simulink model "inverter_switching_GridFollowing_StudentVersion"  (R2025a)
settings: Solver=ode1be  StartTime=0.0  StopTime=0.2  FixedStep=1e-6  MaxStep=1e-7  RelTol=1e-3
values from neighbouring files (symbols this model uses):
  C_Filter = 300e-6    (= 0.0003)    [parameters_StudentVersion.m]
  kFilterIdq = wnFiltreIdq/WnIdq    (= 1)    [parameters_StudentVersion.m]
  kFilterVdq = wnFiltreVdq/WnVdq    (= 1)    [parameters_StudentVersion.m]
  Kpll2 = 1    [parameters_StudentVersion.m]
  L_Filter = 1e-3    (= 0.001)    [parameters_StudentVersion.m]
  rL_filter = 0.1    [parameters_StudentVersion.m]
  T1 = 10/wcpll    (= 10)    [parameters_StudentVersion.m]
  T2 = 1/(10*wcpll)    (= 0.1)    [parameters_StudentVersion.m]
  T32 = sqrt(2/3)*[1 0; -1/2 sqrt(3)/2; -1/2 -sqrt(3)/2]    [parameters_StudentVersion.m]
  Ts = 1/Fs    (= 5e-05)    [parameters_StudentVersion.m]
  Vdc = 800    [parameters_StudentVersion.m]
  Vrms_Grid = 110    [parameters_StudentVersion.m]
  WnIdq = 12000    [parameters_StudentVersion.m]
  WnVdq = 1200    [parameters_StudentVersion.m]
  wrated = 2*pi*60    (= 376.991118431)    [parameters_StudentVersion.m]
  zeta = 1/sqrt(2)    [parameters_StudentVersion.m]
undefined symbols (not defined in the file or in its folder): DiscIntNeverNeededParam
libraries: nesl_utility x22, ee_lib x16, fl_lib x15, simulink x3
(part 1 of 2)
settings Model: Creator=bahrami1  LastModifiedBy=bahrami1

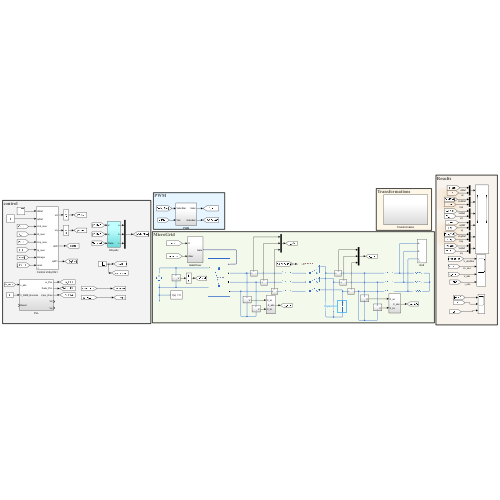
[thumbnail: Simulink's stored preview of the top-level diagram]
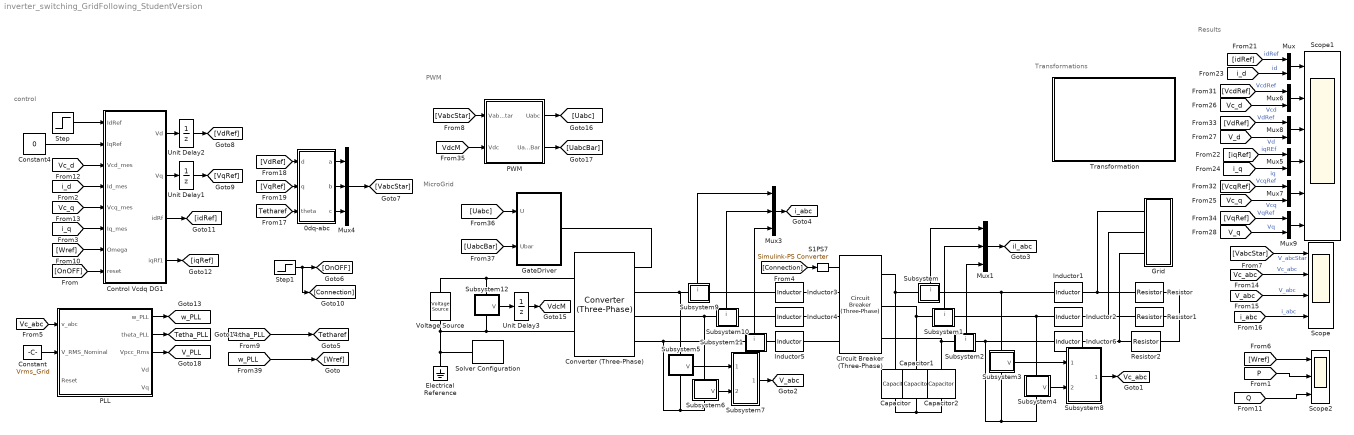
== system inverter_switching_GridFollowing_StudentVersion ==
  note: Transformations
  note: control
  note: MicroGrid
  note: Results
  note: PWM
  0dq-abc : Subsystem
  Capacitor : ee_lib/Passive/Capacitor  cap_option=ee.enum.passive.capacitor.capOption.const  c=10e-6 F  Cvec=[1e-05, 1e-06] F  Vvec=[0, 10] V  CV_table_symmetry=ee.enum.passive.capacitor.tableSymmetry.yes  f_vec=[1, 10] kHz  DFext_vec=[.8, 1.2]  enable_C_tol=ee.enum.toleranceApplication.none  averaging_period=0 s  C_tol=5  tol_distribution=ee.enum.toleranceDistribution.uniform  nSigma=4  r=0 Ohm  g=0 1/Ohm  enable_operating_limits=ee.enum.enable.no  operating_limit_action=ee.enum.passive.reportOpLim.warn  max_working_voltage_range=[-25, 25] V  power_rating=1 W  maxTemperature=85 degC  thermalEnable=false  thermalMass=1 J/K  i_specify=off  i_priority=None  i=0 A  i_nominal_specify=off  i_nominal_value=1  i_nominal_unit=A  v_specify=on  v_priority=None  v=Vrms_Grid*cos(0) V  v_nominal_specify=off  v_nominal_value=1  v_nominal_unit=V  vc_specify=on  vc_priority=High  vc=Vrms_Grid*cos(0) V  vc_nominal_specify=off  vc_nominal_value=1  vc_nominal_unit=V  T_specify=off  T_priority=None  T=298.15 K  T_nominal_specify=off  T_nominal_value=1  T_nominal_unit=K
  Capacitor1 : ee_lib/Passive/Capacitor  cap_option=ee.enum.passive.capacitor.capOption.const  c=10e-6 F  Cvec=[1e-05, 1e-06] F  Vvec=[0, 10] V  CV_table_symmetry=ee.enum.passive.capacitor.tableSymmetry.yes  f_vec=[1, 10] kHz  DFext_vec=[.8, 1.2]  enable_C_tol=ee.enum.toleranceApplication.none  averaging_period=0 s  C_tol=5  tol_distribution=ee.enum.toleranceDistribution.uniform  nSigma=4  r=0 Ohm  g=0 1/Ohm  enable_operating_limits=ee.enum.enable.no  operating_limit_action=ee.enum.passive.reportOpLim.warn  max_working_voltage_range=[-25, 25] V  power_rating=1 W  maxTemperature=85 degC  thermalEnable=false  thermalMass=1 J/K  i_specify=off  i_priority=None  i=0 A  i_nominal_specify=off  i_nominal_value=1  i_nominal_unit=A  v_specify=on  v_priority=None  v=Vrms_Grid*cos(-2*pi/3) V  v_nominal_specify=off  v_nominal_value=1  v_nominal_unit=V  vc_specify=on  vc_priority=High  vc=Vrms_Grid*cos(-2*pi/3) V  vc_nominal_specify=off  vc_nominal_value=1  vc_nominal_unit=V  T_specify=off  T_priority=None  T=298.15 K  T_nominal_specify=off  T_nominal_value=1  T_nominal_unit=K
  Capacitor2 : ee_lib/Passive/Capacitor  cap_option=ee.enum.passive.capacitor.capOption.const  c=10e-6 F  Cvec=[1e-05, 1e-06] F  Vvec=[0, 10] V  CV_table_symmetry=ee.enum.passive.capacitor.tableSymmetry.yes  f_vec=[1, 10] kHz  DFext_vec=[.8, 1.2]  enable_C_tol=ee.enum.toleranceApplication.none  averaging_period=0 s  C_tol=5  tol_distribution=ee.enum.toleranceDistribution.uniform  nSigma=4  r=0 Ohm  g=0 1/Ohm  enable_operating_limits=ee.enum.enable.no  operating_limit_action=ee.enum.passive.reportOpLim.warn  max_working_voltage_range=[-25, 25] V  power_rating=1 W  maxTemperature=85 degC  thermalEnable=false  thermalMass=1 J/K  i_specify=off  i_priority=None  i=0 A  i_nominal_specify=off  i_nominal_value=1  i_nominal_unit=A  v_specify=on  v_priority=None  v=Vrms_Grid*cos(+2*pi/3) V  v_nominal_specify=off  v_nominal_value=1  v_nominal_unit=V  vc_specify=on  vc_priority=High  vc=Vrms_Grid*cos(+2*pi/3) V  vc_nominal_specify=off  vc_nominal_value=1  vc_nominal_unit=V  T_specify=off  T_priority=None  T=298.15 K  T_nominal_specify=off  T_nominal_value=1  T_nominal_unit=K
  Circuit Breaker (Three-Phase) : ee_lib/Switches & Breakers/Circuit Breaker (Three-Phase)  R_closed=1e-9 Ohm  G_open=1e-12 1/Ohm  threshold=0.5 V  breaker_behavior=ee.enum.switches.breakerBehavior.zeroCrossingDisable
      settings: InternalSimscapePortConfiguration="{\"Bottom\":[],\"Left\":[{\"id\":\"vT\",\"label\":\"vT\",\"type\":\"input\"},{\"id\":\"a1\",\"label\":\"a1\",\"type\":\"foundation.electrical.electrical\"},{\"id\":\"b1\",\"label\":\"b1\",\"type\":\"foundation.electrical.electrical\"},{\"id\":\"c1\",\"label\":\"c1\",\"type\":\"foundation.electrical.electrical\"}],\"Right\":[{\"id\":\"a2\",\"label\":\"a2\",\"type\":\"foundation.electrical.electrical\"},{\"id\":\"b2\",\"label\":\"b2\",\"type\":\"foundation.electrical.electrical\"},{\"id\":\"c2\",\"label\":\"c2\",\"type\":\"foundation.electrical.electrical\"}],\"Top\":[]}"
  Constant : Constant  Value=Vrms_Grid
  Constant4 : Constant  Value=0
  Control Vcdq DG1 : Subsystem  mask{rL_DG=rL_filter, L_DG=L_Filter, C_DG=C_Filter, Wn_Idq=WnIdq, kFilter_Idq=kFilterIdq, IntegIdLimitNeg=-30000/L_Filter, IntegIdLimitPos=30000/L_Filter, IntegIqLimitNeg=-30000/L_Filter, IntegIqLimitPos=30000/L_Filter, Wn_Vdq=WnVdq, kFilter_Vdq=kFilterVdq, idRef_Min=-500, idRef_Max=500, iqRef_Min=-500, iqRef_Max=500}
      mask prompts: rL_DG "rl_DG :"; L_DG "L_DG :"; C_DG "C_DG :"; Wn_Idq "Wn_Idq :"; kFilter_Idq "kFilter_Idq :"; Wn_Vdq "Wn_Vdq :"; kFilter_Vdq "kFilter Vdq :"; idRef_Min "idRef_Min :"; idRef_Max "idRef_Max :"; iqRef_Min "iqRef_Min :"; iqRef_Max "iqRef_Max :"
      mask DialogControl ControlGroupParameters Prompt: Control
      mask DialogControl SaturationGroup Prompt: Saturation
  Converter (Three-Phase) : ee_lib/Semiconductors & Converters/Converters/Converter (Three-Phase)  port_option=ee.enum.threePhasePort.expanded  fidelity_option=ee.enum.converters.fidelity.detailed  device_type=ee.enum.converters.switchingdevice.averaged  showThermalPort=false  K=0  Vth=6 V  Vgt=1 V  Vgt_off=-1 V  Ih=1 A  Vf=0.8 V  Ron=0.001 Ohm  Rds=0.001 Ohm  Goff=1e-6 1/Ohm  Eon_scalar=22.86e-3 J  Eoff_scalar=17.14e-3 J  Eoff_natural_commutation=10e-3 J  Voff=300 V  Iout_scalar=600 A  onCurrentMeasDelay=0 s  useCurrentFromPreviousCycle=false  useVoltageFromPreviousCycle=false  diode_param=ee.enum.converters.protectiondiode.chargedynamics  diode_Vf=0.8 V  diode_Ron=0.001 Ohm  diode_Goff=1e-5 1/Ohm  diode_C=50 nF  diode_iRM=-235 A  diode_iF=300 A  diode_idot=-50 A/us  diode_trr_param=ee.enum.converters.diodetrr.trr_factor  diode_trr_factor=3  diode_trr=15 us  diode_Qrr=1500 s*uA  diode_rec_loss_model=ee.enum.diode.reverseRecoveryModel.fixed  diode_ErecVal=0 J  diode_scaleWithIandV=false  diode_ErecMat=zeros(2, 3) J  diode_TjrecVec=[298.15, 398.15] K  diode_IfrecVec=[.1, 1, 10] A  diode_IrecVal=10 A  diode_VrecVal=10 V  diode_tFilter=1 / 1000 / 100 s  thermal_network_parameterization=ee.enum.thermalNetworkTopology.external  Rth=[.08, .5] K/W  Rth_Cauer=[.08, .1, .5] K/W  Rth_Foster=[.08, .14, .22, .16] K/W  thermal_mass_parameterization=ee.enum.thermalNetwork.timeconstant  thermal_mass=[.01, .5] J/K  thermal_mass_Cauer=[.01, .1, .5] J/K  thermal_mass_Foster=[.001, .005, .05, .5] J/K  thermal_time_constant=[.001, .2] s  thermal_time_constant_Cauer=[.001, .1, .2] s  thermal_time_constant_Foster=[7e-05, .0007, .01, .08] s  thermal_mass_initial_temperatures=[25, 25] degC  thermal_mass_initial_temperatures_Cauer=[25, 25, 25] degC  junction_thermal_mass=0.01 J/K  Tvec_initial_Foster=[25, 25, 25, 25] degC  snubber_type=ee.enum.converters.snubber.exclude  Cs=1e-7 F  Rs=0.1 Ohm  Vce_loss=[0, 150, 300] V
      settings: InternalSimscapePortConfiguration="{\"Bottom\":[],\"Left\":[{\"id\":\"G\",\"label\":\"G\",\"type\":\"foundation.electrical.twelve_phase\"},{\"id\":\"a\",\"label\":\"a\",\"type\":\"foundation.electrical.electrical\"},{\"id\":\"b\",\"label\":\"b\",\"type\":\"foundation.electrical.electrical\"},{\"id\":\"c\",\"label\":\"c\",\"type\":\"foundation.electrical.electrical\"}],\"Right\":[{\"id\":\"p\",\"label\":\"+\",\"type\":\"foundation.electrical.electrical\"},{\"id\":\"n\",\"label\":\"-\",\"type\":\"foundation.electrical.electrical\"}],\"Top\":[]}"
  Electrical Reference : fl_lib/Electrical/Electrical Elements/Electrical Reference
  GateDriver : Subsystem
  Grid : Subsystem  mask{Vrms_Grid=Vrms_Grid, F_Grid=60, Phase_Grid=0}
      mask prompts: Vrms_Grid "Grid Voltage (RMS):"; F_Grid "Grid Frequency:"; Phase_Grid "Grid phase angle:"
  Inductor1 : ee_lib/Passive/Inductor  l=1e-3 H  enable_L_tol=ee.enum.toleranceApplication.none  L_tol=20  tol_distribution=ee.enum.toleranceDistribution.uniform  nSigma=4  r=0.5 Ohm  g=1e-9 1/Ohm  enable_operating_limits=ee.enum.enable.no  operating_limit_action=ee.enum.passive.reportOpLim.warn  max_working_current=1 A  power_rating=1 W  i_L_specify=off  i_L_priority=High  i_L=0 A  i_L_nominal_specify=off  i_L_nominal_value=1  i_L_nominal_unit=A
  Inductor2 : ee_lib/Passive/Inductor  l=1e-3 H  enable_L_tol=ee.enum.toleranceApplication.none  L_tol=20  tol_distribution=ee.enum.toleranceDistribution.uniform  nSigma=4  r=0.5 Ohm  g=1e-9 1/Ohm  enable_operating_limits=ee.enum.enable.no  operating_limit_action=ee.enum.passive.reportOpLim.warn  max_working_current=1 A  power_rating=1 W  i_L_specify=off  i_L_priority=High  i_L=0 A  i_L_nominal_specify=off  i_L_nominal_value=1  i_L_nominal_unit=A
  Inductor3 : ee_lib/Passive/Inductor  l=10e-3 H  enable_L_tol=ee.enum.toleranceApplication.none  L_tol=20  tol_distribution=ee.enum.toleranceDistribution.uniform  nSigma=4  r=0 Ohm  g=1e-9 1/Ohm  enable_operating_limits=ee.enum.enable.no  operating_limit_action=ee.enum.passive.reportOpLim.warn  max_working_current=1 A  power_rating=1 W  i_L_specify=off  i_L_priority=High  i_L=0 A  i_L_nominal_specify=off  i_L_nominal_value=1  i_L_nominal_unit=A
  Inductor4 : ee_lib/Passive/Inductor  l=10e-3 H  enable_L_tol=ee.enum.toleranceApplication.none  L_tol=20  tol_distribution=ee.enum.toleranceDistribution.uniform  nSigma=4  r=0 Ohm  g=1e-9 1/Ohm  enable_operating_limits=ee.enum.enable.no  operating_limit_action=ee.enum.passive.reportOpLim.warn  max_working_current=1 A  power_rating=1 W  i_L_specify=off  i_L_priority=High  i_L=0 A  i_L_nominal_specify=off  i_L_nominal_value=1  i_L_nominal_unit=A
  Inductor5 : ee_lib/Passive/Inductor  l=10e-3 H  enable_L_tol=ee.enum.toleranceApplication.none  L_tol=20  tol_distribution=ee.enum.toleranceDistribution.uniform  nSigma=4  r=0 Ohm  g=1e-9 1/Ohm  enable_operating_limits=ee.enum.enable.no  operating_limit_action=ee.enum.passive.reportOpLim.warn  max_working_current=1 A  power_rating=1 W  i_L_specify=off  i_L_priority=High  i_L=0 A  i_L_nominal_specify=off  i_L_nominal_value=1  i_L_nominal_unit=A
  Inductor6 : ee_lib/Passive/Inductor  l=1e-3 H  enable_L_tol=ee.enum.toleranceApplication.none  L_tol=20  tol_distribution=ee.enum.toleranceDistribution.uniform  nSigma=4  r=0.5 Ohm  g=1e-9 1/Ohm  enable_operating_limits=ee.enum.enable.no  operating_limit_action=ee.enum.passive.reportOpLim.warn  max_working_current=1 A  power_rating=1 W  i_L_specify=off  i_L_priority=High  i_L=0 A  i_L_nominal_specify=off  i_L_nominal_value=1  i_L_nominal_unit=A
  Mux{,5..9} (6 alike) : Mux  Inputs=2
  Mux1 : Mux  Inputs=3
  Mux3 : Mux  Inputs=3
  Mux4 : Mux  Inputs=3
  PLL : Subsystem
  PWM : Subsystem
  Resistor : ee_lib/Passive/Resistor  R=5 Ohm  enable_R_tol=ee.enum.toleranceApplication.none  R_tol=5  tol_distribution=ee.enum.toleranceDistribution.uniform  nSigma=4  enable_operating_limits=ee.enum.enable.no  operating_limit_action=ee.enum.passive.reportOpLim.warn  power_rating=1 W  max_working_voltage=100 V  noise_mode=ee.enum.sources.noise.Disabled  Tdevice=25 degC  sample_time=1e-3 s  repeatability=ee.enum.ic.repeatability.notRepeatable  user_seed=0  auto_seed=3890346746  power_derating_T1=70 degC  power_derating_T2=155 degC  operating_temperature_range_vec=[-50, 150] degC  alpha=3.93e-3 1/K  Tmeas=25 degC  thermal_mass=100 J/K  temperature_specify=off  temperature_priority=High  temperature=298.15 K  temperature_nominal_specify=off  temperature_nominal_value=1  temperature_nominal_unit=K
  Resistor1 : ee_lib/Passive/Resistor  R=5 Ohm  enable_R_tol=ee.enum.toleranceApplication.none  R_tol=5  tol_distribution=ee.enum.toleranceDistribution.uniform  nSigma=4  enable_operating_limits=ee.enum.enable.no  operating_limit_action=ee.enum.passive.reportOpLim.warn  power_rating=1 W  max_working_voltage=100 V  noise_mode=ee.enum.sources.noise.Disabled  Tdevice=25 degC  sample_time=1e-3 s  repeatability=ee.enum.ic.repeatability.notRepeatable  user_seed=0  auto_seed=545404223  power_derating_T1=70 degC  power_derating_T2=155 degC  operating_temperature_range_vec=[-50, 150] degC  alpha=3.93e-3 1/K  Tmeas=25 degC  thermal_mass=100 J/K  temperature_specify=off  temperature_priority=High  temperature=298.15 K  temperature_nominal_specify=off  temperature_nominal_value=1  temperature_nominal_unit=K
  Resistor2 : ee_lib/Passive/Resistor  R=5 Ohm  enable_R_tol=ee.enum.toleranceApplication.none  R_tol=5  tol_distribution=ee.enum.toleranceDistribution.uniform  nSigma=4  enable_operating_limits=ee.enum.enable.no  operating_limit_action=ee.enum.passive.reportOpLim.warn  power_rating=1 W  max_working_voltage=100 V  noise_mode=ee.enum.sources.noise.Disabled  Tdevice=25 degC  sample_time=1e-3 s  repeatability=ee.enum.ic.repeatability.notRepeatable  user_seed=0  auto_seed=3922919431  power_derating_T1=70 degC  power_derating_T2=155 degC  operating_temperature_range_vec=[-50, 150] degC  alpha=3.93e-3 1/K  Tmeas=25 degC  thermal_mass=100 J/K  temperature_specify=off  temperature_priority=High  temperature=298.15 K  temperature_nominal_specify=off  temperature_nominal_value=1  temperature_nominal_unit=K
  S1PS7 : nesl_utility/Simulink-PS Converter  PhysicalDomain=network_engine_domain  SubClassName=ps_input  LeftPortType=input  RightPortType=output  PseudoPeriodic=off  Frequencies=[]  NoiseDistribution=none  NoiseParameters=[]  Unit=1  AffineConversion=off  FilteringAndDerivatives=zero  SimscapeFilterOrder=1  InputFilterTimeConstant=.001  UdotUserProvided=1
  Scope : Scope  NumInputPorts=4
      settings: ActiveDisplayString=4  ActiveDisplayYMinimum=-4.8438387041910405  ActiveDisplayYMaximum=5.5775843218677732
  Scope1 : Scope  NumInputPorts=6
      settings: ActiveDisplayString=6  ActiveDisplayYMinimum=-764.96979422436971  ActiveDisplayYMaximum=755.2359372195092
  Scope2 : Scope  NumInputPorts=3
      settings: ActiveDisplayYMinimum=-44.93774115699739  ActiveDisplayYMaximum=222.58045892307609  DataLoggingVariableName=ScopeData2
  Solver Configuration : nesl_utility/Solver Configuration  PhysicalDomain=network_engine_domain  SubClassName=solver  LeftPortType=input  RightPortType=generic  Tones=[]  Harmonics=[]  SimulateNoise=off  Profile=off  UseLocalSampling=off  EnableSwitchedLinearOptims=on  FrequencyDomain=off  UseCCode=off  RelTol=0.001  AbsTol=0.001  MinStep=1e-09  ToWorkspace=off  RevertToSquareIcSolve=off  NumHomotopyIterations=100  PhasorMode=off  PhasorModeNumHarmonics=1  ConsistencySolver=NEWTON_XTOL_AFTER_FTOL  IndexReductionMethod=DerivativeReplacement  DoDC=off  ResidualTolerance=1e-09  ConsistencyTolSource=GLOBAL  ConsistencyAbsTol=0.001  ConsistencyRelTol=0.001  ConsistencyTolFactor=1e-9  UseLocalSolver=off  LocalSolverChoice=NE_PARTITIONING_ADVANCER  ResolveIndetEquations=on  FunctionEvalNumThread=1  LocalSolverSampleTime=50e-6  DoFixedCost=on  MaxNonlinIter=3  MaxModeIter=2  ComputeImpulses=off  ImpulseIterations=2  LinearAlgebra=auto  LinearAlgebraNumThread=0  EquationFormulation=NE_TIME_EF  DelaysMemoryBudget=1024  AutomaticFiltering=on  FilteringTimeConstant=0.001  PartitionStorageMethod=AS_NEEDED  PartitionMemoryBudget=1024  PartitionMethod=ROBUST  MultibodyUseLocalSolver=off  MultibodyLocalSolverChoice=ODE1  MultibodyLocalSolverSampleTime=0.001
  Step : Step  Time=0.04  After=4  SampleTime=0
  Step1 : Step  Time=0.02  Before=1  After=0  SampleTime=0
  Subsystem : Subsystem
      settings: PortSchema="{\"entries\":[{\"content\":{\"sides\":[{\"content\":{\"connectorIds\":[\"LConn1\"]},\"type\":\"ConnectorPlacement.EquallySpacedRectSide\",\"uuid\":\"f9dae77b-82ec-46c0-8ec7-07c4c343cd61\"},{\"content\":{\"connectorIds\":[\"RConn1\"],\"side\":\"RIGHT\"},\"type\":\"ConnectorPlacement.EquallySpacedRectSide\",\"uuid\":\"c868f1e8-59aa-45a3-abdf-5b79dca1cbd6\"},{\"content\":{\"connectorIds\":[\"Out1\"],\"side\":\"TOP\"},\"type\":\"ConnectorPlacement.EquallySpacedRectSide\",\"uuid\":\"1fe3fd4f-ec18-4909-aef2-795910f5eee8\"}]},\"type\":\"ConnectorPlacement.EquallySpacedConnector\",\"uuid\":\"b65f0ac3-40cf-4bf8-a5c1-5ed6a13721a4\"}],\"packageUris\":[\"http://schema.mathworks.com/mf0/Connector/R2020b\"],\"version\":\"1.0\"}"
  Subsystem1 : Subsystem
      settings: PortSchema="{\"entries\":[{\"content\":{\"sides\":[{\"content\":{\"connectorIds\":[\"LConn1\"]},\"type\":\"ConnectorPlacement.EquallySpacedRectSide\",\"uuid\":\"f9dae77b-82ec-46c0-8ec7-07c4c343cd61\"},{\"content\":{\"connectorIds\":[\"RConn1\"],\"side\":\"RIGHT\"},\"type\":\"ConnectorPlacement.EquallySpacedRectSide\",\"uuid\":\"c868f1e8-59aa-45a3-abdf-5b79dca1cbd6\"},{\"content\":{\"connectorIds\":[\"Out1\"],\"side\":\"TOP\"},\"type\":\"ConnectorPlacement.EquallySpacedRectSide\",\"uuid\":\"1fe3fd4f-ec18-4909-aef2-795910f5eee8\"}]},\"type\":\"ConnectorPlacement.EquallySpacedConnector\",\"uuid\":\"b65f0ac3-40cf-4bf8-a5c1-5ed6a13721a4\"}],\"packageUris\":[\"http://schema.mathworks.com/mf0/Connector/R2020b\"],\"version\":\"1.0\"}"
  Subsystem10 : Subsystem
      settings: PortSchema="{\"entries\":[{\"content\":{\"sides\":[{\"content\":{\"connectorIds\":[\"LConn1\"]},\"type\":\"ConnectorPlacement.EquallySpacedRectSide\",\"uuid\":\"f9dae77b-82ec-46c0-8ec7-07c4c343cd61\"},{\"content\":{\"connectorIds\":[\"RConn1\"],\"side\":\"RIGHT\"},\"type\":\"ConnectorPlacement.EquallySpacedRectSide\",\"uuid\":\"c868f1e8-59aa-45a3-abdf-5b79dca1cbd6\"},{\"content\":{\"connectorIds\":[\"Out1\"],\"side\":\"TOP\"},\"type\":\"ConnectorPlacement.EquallySpacedRectSide\",\"uuid\":\"1fe3fd4f-ec18-4909-aef2-795910f5eee8\"}]},\"type\":\"ConnectorPlacement.EquallySpacedConnector\",\"uuid\":\"b65f0ac3-40cf-4bf8-a5c1-5ed6a13721a4\"}],\"packageUris\":[\"http://schema.mathworks.com/mf0/Connector/R2020b\"],\"version\":\"1.0\"}"
  Subsystem11 : Subsystem
      settings: PortSchema="{\"entries\":[{\"content\":{\"sides\":[{\"content\":{\"connectorIds\":[\"LConn1\"]},\"type\":\"ConnectorPlacement.EquallySpacedRectSide\",\"uuid\":\"f9dae77b-82ec-46c0-8ec7-07c4c343cd61\"},{\"content\":{\"connectorIds\":[\"RConn1\"],\"side\":\"RIGHT\"},\"type\":\"ConnectorPlacement.EquallySpacedRectSide\",\"uuid\":\"c868f1e8-59aa-45a3-abdf-5b79dca1cbd6\"},{\"content\":{\"connectorIds\":[\"Out1\"],\"side\":\"TOP\"},\"type\":\"ConnectorPlacement.EquallySpacedRectSide\",\"uuid\":\"1fe3fd4f-ec18-4909-aef2-795910f5eee8\"}]},\"type\":\"ConnectorPlacement.EquallySpacedConnector\",\"uuid\":\"b65f0ac3-40cf-4bf8-a5c1-5ed6a13721a4\"}],\"packageUris\":[\"http://schema.mathworks.com/mf0/Connector/R2020b\"],\"version\":\"1.0\"}"
  Subsystem12 : Subsystem
      settings: PortSchema="{\"entries\":[{\"content\":{\"sides\":[{\"content\":{},\"type\":\"ConnectorPlacement.EquallySpacedRectSide\",\"uuid\":\"f9dae77b-82ec-46c0-8ec7-07c4c343cd61\"},{\"content\":{\"connectorIds\":[\"Out1\"],\"side\":\"RIGHT\"},\"type\":\"ConnectorPlacement.EquallySpacedRectSide\",\"uuid\":\"c868f1e8-59aa-45a3-abdf-5b79dca1cbd6\"},{\"content\":{\"connectorIds\":[\"LConn1\"],\"side\":\"TOP\"},\"type\":\"ConnectorPlacement.EquallySpacedRectSide\",\"uuid\":\"1fe3fd4f-ec18-4909-aef2-795910f5eee8\"},{\"content\":{\"connectorIds\":[\"RConn1\"],\"side\":\"BOTTOM\"},\"type\":\"ConnectorPlacement.EquallySpacedRectSide\",\"uuid\":\"67a88f15-4497-4048-9449-885deab38afe\"}]},\"type\":\"ConnectorPlacement.EquallySpacedConnector\",\"uuid\":\"b65f0ac3-40cf-4bf8-a5c1-5ed6a13721a4\"}],\"packageUris\":[\"http://schema.mathworks.com/mf0/Connector/R2020b\"],\"version\":\"1.0\"}"
  Subsystem2 : Subsystem
      settings: PortSchema="{\"entries\":[{\"content\":{\"sides\":[{\"content\":{\"connectorIds\":[\"LConn1\"]},\"type\":\"ConnectorPlacement.EquallySpacedRectSide\",\"uuid\":\"f9dae77b-82ec-46c0-8ec7-07c4c343cd61\"},{\"content\":{\"connectorIds\":[\"RConn1\"],\"side\":\"RIGHT\"},\"type\":\"ConnectorPlacement.EquallySpacedRectSide\",\"uuid\":\"c868f1e8-59aa-45a3-abdf-5b79dca1cbd6\"},{\"content\":{\"connectorIds\":[\"Out1\"],\"side\":\"TOP\"},\"type\":\"ConnectorPlacement.EquallySpacedRectSide\",\"uuid\":\"1fe3fd4f-ec18-4909-aef2-795910f5eee8\"}]},\"type\":\"ConnectorPlacement.EquallySpacedConnector\",\"uuid\":\"b65f0ac3-40cf-4bf8-a5c1-5ed6a13721a4\"}],\"packageUris\":[\"http://schema.mathworks.com/mf0/Connector/R2020b\"],\"version\":\"1.0\"}"
  Subsystem3 : Subsystem
      settings: PortSchema="{\"entries\":[{\"content\":{\"sides\":[{\"content\":{},\"type\":\"ConnectorPlacement.EquallySpacedRectSide\",\"uuid\":\"f9dae77b-82ec-46c0-8ec7-07c4c343cd61\"},{\"content\":{\"connectorIds\":[\"Out1\"],\"side\":\"RIGHT\"},\"type\":\"ConnectorPlacement.EquallySpacedRectSide\",\"uuid\":\"c868f1e8-59aa-45a3-abdf-5b79dca1cbd6\"},{\"content\":{\"connectorIds\":[\"LConn1\"],\"side\":\"TOP\"},\"type\":\"ConnectorPlacement.EquallySpacedRectSide\",\"uuid\":\"1fe3fd4f-ec18-4909-aef2-795910f5eee8\"},{\"content\":{\"connectorIds\":[\"RConn1\"],\"side\":\"BOTTOM\"},\"type\":\"ConnectorPlacement.EquallySpacedRectSide\",\"uuid\":\"67a88f15-4497-4048-9449-885deab38afe\"}]},\"type\":\"ConnectorPlacement.EquallySpacedConnector\",\"uuid\":\"b65f0ac3-40cf-4bf8-a5c1-5ed6a13721a4\"}],\"packageUris\":[\"http://schema.mathworks.com/mf0/Connector/R2020b\"],\"version\":\"1.0\"}"
  Subsystem4 : Subsystem
      settings: PortSchema="{\"entries\":[{\"content\":{\"sides\":[{\"content\":{},\"type\":\"ConnectorPlacement.EquallySpacedRectSide\",\"uuid\":\"f9dae77b-82ec-46c0-8ec7-07c4c343cd61\"},{\"content\":{\"connectorIds\":[\"Out1\"],\"side\":\"RIGHT\"},\"type\":\"ConnectorPlacement.EquallySpacedRectSide\",\"uuid\":\"c868f1e8-59aa-45a3-abdf-5b79dca1cbd6\"},{\"content\":{\"connectorIds\":[\"LConn1\"],\"side\":\"TOP\"},\"type\":\"ConnectorPlacement.EquallySpacedRectSide\",\"uuid\":\"1fe3fd4f-ec18-4909-aef2-795910f5eee8\"},{\"content\":{\"connectorIds\":[\"RConn1\"],\"side\":\"BOTTOM\"},\"type\":\"ConnectorPlacement.EquallySpacedRectSide\",\"uuid\":\"67a88f15-4497-4048-9449-885deab38afe\"}]},\"type\":\"ConnectorPlacement.EquallySpacedConnector\",\"uuid\":\"b65f0ac3-40cf-4bf8-a5c1-5ed6a13721a4\"}],\"packageUris\":[\"http://schema.mathworks.com/mf0/Connector/R2020b\"],\"version\":\"1.0\"}"
  Subsystem5 : Subsystem
      settings: PortSchema="{\"entries\":[{\"content\":{\"sides\":[{\"content\":{},\"type\":\"ConnectorPlacement.EquallySpacedRectSide\",\"uuid\":\"f9dae77b-82ec-46c0-8ec7-07c4c343cd61\"},{\"content\":{\"connectorIds\":[\"Out1\"],\"side\":\"RIGHT\"},\"type\":\"ConnectorPlacement.EquallySpacedRectSide\",\"uuid\":\"c868f1e8-59aa-45a3-abdf-5b79dca1cbd6\"},{\"content\":{\"connectorIds\":[\"LConn1\"],\"side\":\"TOP\"},\"type\":\"ConnectorPlacement.EquallySpacedRectSide\",\"uuid\":\"1fe3fd4f-ec18-4909-aef2-795910f5eee8\"},{\"content\":{\"connectorIds\":[\"RConn1\"],\"side\":\"BOTTOM\"},\"type\":\"ConnectorPlacement.EquallySpacedRectSide\",\"uuid\":\"67a88f15-4497-4048-9449-885deab38afe\"}]},\"type\":\"ConnectorPlacement.EquallySpacedConnector\",\"uuid\":\"b65f0ac3-40cf-4bf8-a5c1-5ed6a13721a4\"}],\"packageUris\":[\"http://schema.mathworks.com/mf0/Connector/R2020b\"],\"version\":\"1.0\"}"
  Subsystem6 : Subsystem
      settings: PortSchema="{\"entries\":[{\"content\":{\"sides\":[{\"content\":{},\"type\":\"ConnectorPlacement.EquallySpacedRectSide\",\"uuid\":\"f9dae77b-82ec-46c0-8ec7-07c4c343cd61\"},{\"content\":{\"connectorIds\":[\"Out1\"],\"side\":\"RIGHT\"},\"type\":\"ConnectorPlacement.EquallySpacedRectSide\",\"uuid\":\"c868f1e8-59aa-45a3-abdf-5b79dca1cbd6\"},{\"content\":{\"connectorIds\":[\"LConn1\"],\"side\":\"TOP\"},\"type\":\"ConnectorPlacement.EquallySpacedRectSide\",\"uuid\":\"1fe3fd4f-ec18-4909-aef2-795910f5eee8\"},{\"content\":{\"connectorIds\":[\"RConn1\"],\"side\":\"BOTTOM\"},\"type\":\"ConnectorPlacement.EquallySpacedRectSide\",\"uuid\":\"67a88f15-4497-4048-9449-885deab38afe\"}]},\"type\":\"ConnectorPlacement.EquallySpacedConnector\",\"uuid\":\"b65f0ac3-40cf-4bf8-a5c1-5ed6a13721a4\"}],\"packageUris\":[\"http://schema.mathworks.com/mf0/Connector/R2020b\"],\"version\":\"1.0\"}"
  Subsystem7 : Subsystem
  Subsystem8 : Subsystem
  Subsystem9 : Subsystem
      settings: PortSchema="{\"entries\":[{\"content\":{\"sides\":[{\"content\":{\"connectorIds\":[\"LConn1\"]},\"type\":\"ConnectorPlacement.EquallySpacedRectSide\",\"uuid\":\"f9dae77b-82ec-46c0-8ec7-07c4c343cd61\"},{\"content\":{\"connectorIds\":[\"RConn1\"],\"side\":\"RIGHT\"},\"type\":\"ConnectorPlacement.EquallySpacedRectSide\",\"uuid\":\"c868f1e8-59aa-45a3-abdf-5b79dca1cbd6\"},{\"content\":{\"connectorIds\":[\"Out1\"],\"side\":\"TOP\"},\"type\":\"ConnectorPlacement.EquallySpacedRectSide\",\"uuid\":\"1fe3fd4f-ec18-4909-aef2-795910f5eee8\"}]},\"type\":\"ConnectorPlacement.EquallySpacedConnector\",\"uuid\":\"b65f0ac3-40cf-4bf8-a5c1-5ed6a13721a4\"}],\"packageUris\":[\"http://schema.mathworks.com/mf0/Connector/R2020b\"],\"version\":\"1.0\"}"
  Transformation : Subsystem
  Unit Delay1 : UnitDelay  SampleTime=-1  HasFrameUpgradeWarning=on
  Unit Delay2 : UnitDelay  SampleTime=-1  HasFrameUpgradeWarning=on
  Unit Delay3 : UnitDelay  InitialCondition=Vdc  SampleTime=-1  HasFrameUpgradeWarning=on
  Voltage Source : ee_lib/Sources/Voltage Source  dc_voltage=Vdc V  ac_voltage=0 V  ac_shift=0 rad  ac_frequency=50 Hz  noise_mode=ee.enum.sources.noise.Disabled  PSD=0 V^2/Hz  sample_time=1e-3 s  repeatability=ee.enum.sources.repeatability.NotRepeatable  user_seed=0  auto_seed=2715962282  i_specify=off  i_priority=None  i=0 A  i_nominal_specify=off  i_nominal_value=1  i_nominal_unit=A  v_specify=off  v_priority=None  v=0 V  v_nominal_specify=off  v_nominal_value=1  v_nominal_unit=V
  tag scope: Tetha_PLL=global, Tetharef=global, V_PLL=global, V_abc=global, Vc_abc=global, VdcM=global, i_abc=global, il_abc=global, w_PLL=global
  wires:
  Subsystem/1(i) -> Mux1/1
  Subsystem1/1(i) -> Mux1/2
  Subsystem2/1(i) -> Mux1/3
  [VabcStar] -> Scope/1  "V_abcStar"
  Mux4/1 -> [VabcStar]
  Subsystem6/1(V) -> Subsystem7/2(X_bc)
  Subsystem5/1(V) -> Subsystem7/1(X_ac)
  Subsystem3/1(V) -> Subsystem8/1(X_ac)
  Subsystem4/1(V) -> Subsystem8/2(X_bc)
  Subsystem7/1(X_abc) -> [V_abc]
  Subsystem8/1(X_abc) -> [Vc_abc]
  Mux1/1 -> [il_abc]
  Subsystem11/1(i) -> Mux3/3
  Subsystem10/1(i) -> Mux3/2
  Subsystem9/1(i) -> Mux3/1
  Mux3/1 -> [i_abc]
  [Vc_d] -> Control Vcdq DG1/3(Vcd_mes)
  [Vc_q] -> Control Vcdq DG1/5(Vcq_mes)
  [i_d] -> Control Vcdq DG1/4(Id_mes)
  [i_q] -> Control Vcdq DG1/6(Iq_mes)
  [Wref] -> Control Vcdq DG1/7(Omega)
  [Vc_abc] -> Scope/2  "Vc_abc"
  [V_abc] -> Scope/3  "V_abc"
  [i_abc] -> Scope/4  "i_abc"
  Control Vcdq DG1/1(Vd) -> Unit Delay2/1
  Control Vcdq DG1/2(Vq) -> Unit Delay1/1
  0dq-abc/1(a) -> Mux4/1
  0dq-abc/2(b) -> Mux4/2
  0dq-abc/3(c) -> Mux4/3
  [Tetharef] -> 0dq-abc/3(theta)
  [VdRef] -> 0dq-abc/1(d)
  [VqRef] -> 0dq-abc/2(q)
  Unit Delay2/1 -> [VdRef]
  Unit Delay1/1 -> [VqRef]
  Control Vcdq DG1/3(idRf) -> [idRef]
  Control Vcdq DG1/4(iqRf1) -> [iqRef]
  [i_d] -> Mux/2  "id"
  [idRef] -> Mux/1  "idRef"
  Mux/1 -> Scope1/1
  [iqRef] -> Mux5/1  "iqREf"
  [i_q] -> Mux5/2  "iq"
  [VcdRef] -> Mux6/1  "VcdRef"
  [Vc_d] -> Mux6/2  "Vcd"
  [VcqRef] -> Mux7/1  "VcqRef"
  [Vc_q] -> Mux7/2  "Vcq"
  Mux9/1 -> Scope1/6
  [VdRef] -> Mux8/1  "VdRef"
  [V_d] -> Mux8/2  "Vd"
  [V_q] -> Mux9/2  "Vq"
  [VqRef] -> Mux9/1  "VqRef"
  Mux5/1 -> Scope1/4
  Mux6/1 -> Scope1/2
  Mux8/1 -> Scope1/3
  Mux7/1 -> Scope1/5
  [VabcStar] -> PWM/1(VabcStar)
  Subsystem12/1(V) -> Unit Delay3/1
  [VdcM] -> PWM/2(Vdc)
  PWM/1(Uabc) -> [Uabc]
  PWM/2(UabcBar) -> [UabcBar]
  [Uabc] -> GateDriver/1(U)
  [UabcBar] -> GateDriver/2(Ubar)
  Unit Delay3/1 -> [VdcM]
  [OnOFF] -> Control Vcdq DG1/8(reset)
  [Connection] -> S1PS7/1
  [Vc_abc] -> PLL/1(v_abc)
  Constant/1 -> PLL/2(V_RMS_Nominal)
  [Wref] -> Scope2/1
  PLL/3(Vpcc_Rms) -> [V_PLL]
  PLL/2(theta_PLL) -> [Tetha_PLL]
  PLL/1(w_PLL) -> [w_PLL]
  [w_PLL] -> [Wref]
  Step/1 -> Control Vcdq DG1/1(IdRef)
  Constant4/1 -> Control Vcdq DG1/2(IqRef)
  [P] -> Scope2/2
  [Q] -> Scope2/3
  [Tetha_PLL] -> [Tetharef]
  Step1/1 -> [Connection], [OnOFF]
  connections:
  Voltage Source/RConn1 -- Converter (Three-Phase)/RConn2 -- Subsystem12/RConn1 -- Solver Configuration/RConn1 -- Electrical Reference/LConn1
  Resistor/RConn1 -- Resistor1/RConn1 -- Resistor2/RConn1
  Subsystem/RConn1 -- Inductor1/LConn1 -- Subsystem3/LConn1
  Subsystem9/RConn1 -- Inductor3/LConn1
  Capacitor/LConn1 -- Circuit Breaker (Three-Phase)/RConn1 -- Subsystem/LConn1
  Inductor4/LConn1 -- Subsystem10/RConn1
  Subsystem5/RConn1 -- Converter (Three-Phase)/LConn4 -- Subsystem11/LConn1 -- Subsystem6/RConn1
  Subsystem1/LConn1 -- Capacitor1/LConn1 -- Circuit Breaker (Three-Phase)/RConn2
  Subsystem2/LConn1 -- Capacitor2/LConn1 -- Circuit Breaker (Three-Phase)/RConn3
  Capacitor/RConn1 -- Capacitor2/RConn1 -- Capacitor1/RConn1
  Converter (Three-Phase)/RConn1 -- Subsystem12/LConn1 -- Voltage Source/LConn1
  Subsystem5/LConn1 -- Converter (Three-Phase)/LConn2 -- Subsystem9/LConn1
  Subsystem6/LConn1 -- Subsystem10/LConn1 -- Converter (Three-Phase)/LConn3
  Inductor5/LConn1 -- Subsystem11/RConn1
  GateDriver/RConn1 -- Converter (Three-Phase)/LConn1
  S1PS7/RConn1 -- Circuit Breaker (Three-Phase)/LConn1
  Circuit Breaker (Three-Phase)/LConn2 -- Inductor3/RConn1
  Inductor4/RConn1 -- Circuit Breaker (Three-Phase)/LConn3
  Inductor5/RConn1 -- Circuit Breaker (Three-Phase)/LConn4
  Resistor1/LConn1 -- Inductor2/RConn1 -- Grid/LConn2
  Resistor2/LConn1 -- Inductor6/RConn1 -- Grid/LConn3
  Subsystem2/RConn1 -- Inductor6/LConn1 -- Subsystem3/RConn1 -- Subsystem4/RConn1
  Subsystem1/RConn1 -- Inductor2/LConn1 -- Subsystem4/LConn1
  Resistor/LConn1 -- Inductor1/RConn1 -- Grid/LConn1

== system inverter_switching_GridFollowing_StudentVersion/0dq-abc ==
  d : Inport
  q : Inport  Port=2
  theta : Inport  Port=3
  Fcn1 : Fcn  Expr=sqrt(2/3)*(u[1]/sqrt(2)+u[2]*cos(u[4]-2*pi/3)-u[3]*sin(u[4]-2*pi/3))
  Fcn2 : Fcn  Expr=sqrt(2/3)*(u[1]/sqrt(2)+u[2]*cos(u[4]-4*pi/3)-u[3]*sin(u[4]-4*pi/3))
  Fcn3 : Fcn  Expr=sqrt(2/3)*(u[1]/sqrt(2)+u[2]*cos(u[4])-u[3]*sin(u[4]))
  Mux2 : Mux
  a : Outport  InitialOutput=0
  b : Outport  Port=2  InitialOutput=0
  c : Outport  Port=3  InitialOutput=0
  wires:
  Fcn2/1 -> c/1
  Fcn1/1 -> b/1
  Fcn3/1 -> a/1
  q/1 -> Mux2/3
  d/1 -> Mux2/2
  theta/1 -> Mux2/4
  Mux2/1 -> Fcn3/1, Fcn2/1, Fcn1/1

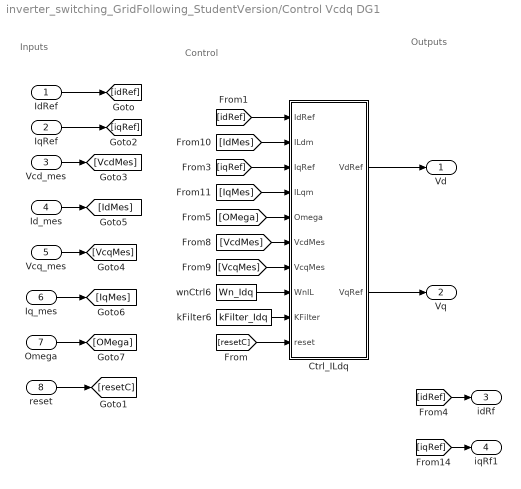
== system inverter_switching_GridFollowing_StudentVersion/Control Vcdq DG1 ==
  note: Outputs
  note: Control
  note: Inputs
  IdRef : Inport
  IqRef : Inport  Port=2
  Vcd_mes : Inport  Port=3
  Id_mes : Inport  Port=4
  Vcq_mes : Inport  Port=5
  Iq_mes : Inport  Port=6
  Omega : Inport  Port=7
  reset : Inport  Port=8
  Ctrl_ILdq : Subsystem
  kFilter6 : Constant  Value=kFilter_Idq
  wnCtrl6 : Constant  Value=Wn_Idq
  Vd : Outport
  Vq : Outport  Port=2
  idRf : Outport  Port=3
  iqRf1 : Outport  Port=4
  wires:
  [idRef] -> Ctrl_ILdq/1(IdRef)
  wnCtrl6/1 -> Ctrl_ILdq/8(WnIL)
  kFilter6/1 -> Ctrl_ILdq/9(KFilter)
  [VcqMes] -> Ctrl_ILdq/7(VcqMes)
  [VcdMes] -> Ctrl_ILdq/6(VcdMes)
  [resetC] -> Ctrl_ILdq/10(reset)
  Ctrl_ILdq/2(VqRef) -> Vq/1
  Ctrl_ILdq/1(VdRef) -> Vd/1
  reset/1 -> [resetC]
  [iqRef] -> Ctrl_ILdq/3(IqRef)
  Vcd_mes/1 -> [VcdMes]
  Vcq_mes/1 -> [VcqMes]
  Id_mes/1 -> [IdMes]
  [IdMes] -> Ctrl_ILdq/2(ILdm)
  Iq_mes/1 -> [IqMes]
  [IqMes] -> Ctrl_ILdq/4(ILqm)
  Omega/1 -> [OMega]
  [OMega] -> Ctrl_ILdq/5(Omega)
  [iqRef] -> iqRf1/1
  [idRef] -> idRf/1
  IdRef/1 -> [idRef]
  IqRef/1 -> [iqRef]

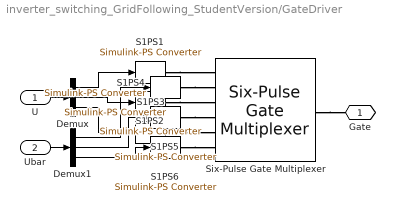
== system inverter_switching_GridFollowing_StudentVersion/GateDriver ==
  U : Inport
  Ubar : Inport  Port=2
  Demux : Demux  Outputs=3
  Demux1 : Demux  Outputs=3
  S1PS{1..6} (6 alike) : nesl_utility/Simulink-PS Converter  PhysicalDomain=network_engine_domain  SubClassName=ps_input  LeftPortType=input  RightPortType=output  PseudoPeriodic=off  Frequencies=[]  NoiseDistribution=none  NoiseParameters=[]  Unit=1  AffineConversion=off  FilteringAndDerivatives=zero  SimscapeFilterOrder=1  InputFilterTimeConstant=.001  UdotUserProvided=1
  Six-Pulse Gate Multiplexer : ee_lib/Semiconductors & Converters/Converters/Six-Pulse Gate Multiplexer  port_option=ee.enum.controlport.ps
  Gate : PMIOPort  Side=Right
  wires:
  Demux/2 -> S1PS2/1
  Demux1/3 -> S1PS6/1
  Demux/3 -> S1PS3/1
  Demux1/1 -> S1PS4/1
  Demux1/2 -> S1PS5/1
  Demux/1 -> S1PS1/1
  Ubar/1 -> Demux1/1
  U/1 -> Demux/1
  connections:
  S1PS3/RConn1 -- Six-Pulse Gate Multiplexer/LConn5
  S1PS6/RConn1 -- Six-Pulse Gate Multiplexer/LConn6
  S1PS5/RConn1 -- Six-Pulse Gate Multiplexer/LConn4
  S1PS2/RConn1 -- Six-Pulse Gate Multiplexer/LConn3
  S1PS1/RConn1 -- Six-Pulse Gate Multiplexer/LConn1
  S1PS4/RConn1 -- Six-Pulse Gate Multiplexer/LConn2
  Six-Pulse Gate Multiplexer/RConn1 -- Gate/RConn1

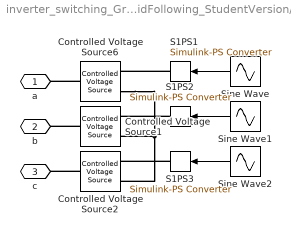
== system inverter_switching_GridFollowing_StudentVersion/Grid ==
  Controlled Voltage Source1 : fl_lib/Electrical/Electrical Sources/Controlled Voltage Source
  Controlled Voltage Source2 : fl_lib/Electrical/Electrical Sources/Controlled Voltage Source
  Controlled Voltage Source6 : fl_lib/Electrical/Electrical Sources/Controlled Voltage Source
  S1PS1 : nesl_utility/Simulink-PS Converter  PhysicalDomain=network_engine_domain  SubClassName=ps_input  LeftPortType=input  RightPortType=output  PseudoPeriodic=off  Frequencies=[]  NoiseDistribution=none  NoiseParameters=[]  Unit=1  AffineConversion=off  FilteringAndDerivatives=zero  SimscapeFilterOrder=1  InputFilterTimeConstant=.001  UdotUserProvided=1
  S1PS2 : nesl_utility/Simulink-PS Converter  PhysicalDomain=network_engine_domain  SubClassName=ps_input  LeftPortType=input  RightPortType=output  PseudoPeriodic=off  Frequencies=[]  NoiseDistribution=none  NoiseParameters=[]  Unit=1  AffineConversion=off  FilteringAndDerivatives=zero  SimscapeFilterOrder=1  InputFilterTimeConstant=.001  UdotUserProvided=1
  S1PS3 : nesl_utility/Simulink-PS Converter  PhysicalDomain=network_engine_domain  SubClassName=ps_input  LeftPortType=input  RightPortType=output  PseudoPeriodic=off  Frequencies=[]  NoiseDistribution=none  NoiseParameters=[]  Unit=1  AffineConversion=off  FilteringAndDerivatives=zero  SimscapeFilterOrder=1  InputFilterTimeConstant=.001  UdotUserProvided=1
  Sine Wave : Sin  Amplitude=Vrms_Grid*sqrt(2)  Frequency=F_Grid  Phase=Phase_Grid+pi/2
  Sine Wave1 : Sin  Amplitude=Vrms_Grid*sqrt(2)  Frequency=F_Grid  Phase=Phase_Grid-2*pi/3+pi/2
  Sine Wave2 : Sin  Amplitude=Vrms_Grid*sqrt(2)  Frequency=F_Grid  Phase=Phase_Grid+2*pi/3+pi/2
  a : PMIOPort  Side=Left
  b : PMIOPort  Port=2  Side=Left
  c : PMIOPort  Port=3  Side=Left
  wires:
  Sine Wave/1 -> S1PS1/1
  Sine Wave1/1 -> S1PS2/1
  Sine Wave2/1 -> S1PS3/1
  connections:
  Controlled Voltage Source1/RConn2 -- Controlled Voltage Source2/RConn2 -- Controlled Voltage Source6/RConn2
  S1PS3/RConn1 -- Controlled Voltage Source2/RConn1
  S1PS1/RConn1 -- Controlled Voltage Source6/RConn1
  S1PS2/RConn1 -- Controlled Voltage Source1/RConn1
  Controlled Voltage Source2/LConn1 -- c/RConn1
  Controlled Voltage Source1/LConn1 -- b/RConn1
  Controlled Voltage Source6/LConn1 -- a/RConn1

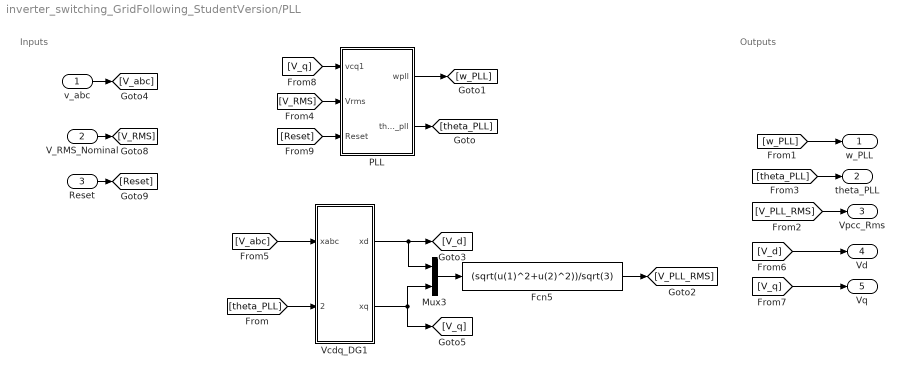
== system inverter_switching_GridFollowing_StudentVersion/PLL ==
  note: Outputs
  note: Inputs
  v_abc : Inport
  V_RMS_Nominal : Inport  Port=2
  Reset : Inport  Port=3
  Fcn5 : Fcn  Expr=(sqrt(u(1)^2+u(2)^2))/sqrt(3)
  Mux3 : Mux  Inputs=2
  PLL : Subsystem
  Vcdq_DG1 : Subsystem
  w_PLL : Outport
  theta_PLL : Outport  Port=2
  Vpcc_Rms : Outport  Port=3
  Vd : Outport  Port=4
  Vq : Outport  Port=5
  wires:
  Mux3/1 -> Fcn5/1
  Vcdq_DG1/1(xd) -> [V_d], Mux3/1
  Vcdq_DG1/2(xq) -> [V_q], Mux3/2
  [theta_PLL] -> Vcdq_DG1/2(theta_pll)
  PLL/2(theta_pll) -> [theta_PLL]
  PLL/1(wpll) -> [w_PLL]
  [w_PLL] -> w_PLL/1
  Fcn5/1 -> [V_PLL_RMS]
  [V_PLL_RMS] -> Vpcc_Rms/1
  [theta_PLL] -> theta_PLL/1
  [V_q] -> PLL/1(vcq1)
  v_abc/1 -> [V_abc]
  V_RMS_Nominal/1 -> [V_RMS]
  [V_RMS] -> PLL/2(Vrms)
  Reset/1 -> [Reset]
  [Reset] -> PLL/3(Reset)
  [V_d] -> Vd/1
  [V_q] -> Vq/1
  [V_abc] -> Vcdq_DG1/1(xabc)

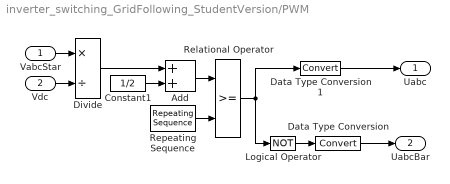
== system inverter_switching_GridFollowing_StudentVersion/PWM ==
  VabcStar : Inport
  Vdc : Inport  Port=2
  Add : Sum
  Constant1 : Constant  Value=1/2
  Data Type Conversion : DataTypeConversion  SaturateOnIntegerOverflow=off  RndMeth=Floor
  Data Type Conversion1 : DataTypeConversion  SaturateOnIntegerOverflow=off  RndMeth=Floor
  Divide : Product  Inputs=*/
  Logical Operator : Logic  Operator=NOT  AllPortsSameDT=off  OutDataTypeStr=boolean
  Relational Operator : RelationalOperator  OutDataTypeStr=boolean  RndMeth=Simplest  InputSameDT=off
  Repeating Sequence : simulink/Sources/Repeating Sequence  rep_seq_t=[0 1/2 1]*Ts  rep_seq_y=[0 1 0]
  Uabc : Outport
  UabcBar : Outport  Port=2
  wires:
  Divide/1 -> Add/1
  Relational Operator/1 -> Logical Operator/1, Data Type Conversion1/1
  Vdc/1 -> Divide/2
  Add/1 -> Relational Operator/1
  Constant1/1 -> Add/2
  Logical Operator/1 -> Data Type Conversion/1
  Data Type Conversion1/1 -> Uabc/1
  VabcStar/1 -> Divide/1
  Repeating Sequence/1 -> Relational Operator/2
  Data Type Conversion/1 -> UabcBar/1

== system inverter_switching_GridFollowing_StudentVersion/Subsystem ==
  Current Sensor : fl_lib/Electrical/Electrical Sensors/Current Sensor
  PS-Simulink Converter : nesl_utility/PS-Simulink Converter  PhysicalDomain=network_engine_domain  SubClassName=ps_output  LeftPortType=input  RightPortType=output  PseudoPeriodic=off  Frequencies=[]  VectorFormat=inherit  Unit=inherit  AffineConversion=off
  + : PMIOPort  Side=Left
  - : PMIOPort  Port=2  Side=Right
  i : Outport
  wires:
  PS-Simulink Converter/1 -> i/1
  connections:
  PS-Simulink Converter/LConn1 -- Current Sensor/RConn1
  Current Sensor/LConn1 -- +/RConn1
  Current Sensor/RConn2 -- -/RConn1

== system inverter_switching_GridFollowing_StudentVersion/Subsystem1 ==
  Current Sensor : fl_lib/Electrical/Electrical Sensors/Current Sensor
  PS-Simulink Converter : nesl_utility/PS-Simulink Converter  PhysicalDomain=network_engine_domain  SubClassName=ps_output  LeftPortType=input  RightPortType=output  PseudoPeriodic=off  Frequencies=[]  VectorFormat=inherit  Unit=inherit  AffineConversion=off
  + : PMIOPort  Side=Left
  - : PMIOPort  Port=2  Side=Right
  i : Outport
  wires:
  PS-Simulink Converter/1 -> i/1
  connections:
  Current Sensor/RConn2 -- -/RConn1
  Current Sensor/LConn1 -- +/RConn1
  PS-Simulink Converter/LConn1 -- Current Sensor/RConn1

== system inverter_switching_GridFollowing_StudentVersion/Subsystem10 ==
  Current Sensor : fl_lib/Electrical/Electrical Sensors/Current Sensor
  PS-Simulink Converter : nesl_utility/PS-Simulink Converter  PhysicalDomain=network_engine_domain  SubClassName=ps_output  LeftPortType=input  RightPortType=output  PseudoPeriodic=off  Frequencies=[]  VectorFormat=inherit  Unit=inherit  AffineConversion=off
  + : PMIOPort  Side=Left
  - : PMIOPort  Port=2  Side=Right
  i : Outport
  wires:
  PS-Simulink Converter/1 -> i/1
  connections:
  PS-Simulink Converter/LConn1 -- Current Sensor/RConn1
  Current Sensor/LConn1 -- +/RConn1
  Current Sensor/RConn2 -- -/RConn1

== system inverter_switching_GridFollowing_StudentVersion/Subsystem11 ==
  Current Sensor : fl_lib/Electrical/Electrical Sensors/Current Sensor
  PS-Simulink Converter : nesl_utility/PS-Simulink Converter  PhysicalDomain=network_engine_domain  SubClassName=ps_output  LeftPortType=input  RightPortType=output  PseudoPeriodic=off  Frequencies=[]  VectorFormat=inherit  Unit=inherit  AffineConversion=off
  + : PMIOPort  Side=Left
  - : PMIOPort  Port=2  Side=Right
  i : Outport
  wires:
  PS-Simulink Converter/1 -> i/1
  connections:
  Current Sensor/RConn2 -- -/RConn1
  Current Sensor/LConn1 -- +/RConn1
  PS-Simulink Converter/LConn1 -- Current Sensor/RConn1

== system inverter_switching_GridFollowing_StudentVersion/Subsystem12 ==
  PS-Simulink Converter : nesl_utility/PS-Simulink Converter  PhysicalDomain=network_engine_domain  SubClassName=ps_output  LeftPortType=input  RightPortType=output  PseudoPeriodic=off  Frequencies=[]  VectorFormat=inherit  Unit=inherit  AffineConversion=off
  Voltage Sensor : fl_lib/Electrical/Electrical Sensors/Voltage Sensor
  + : PMIOPort  Side=Left
  - : PMIOPort  Port=2  Side=Right
  V : Outport
  wires:
  PS-Simulink Converter/1 -> V/1
  connections:
  Voltage Sensor/RConn2 -- -/RConn1
  PS-Simulink Converter/LConn1 -- Voltage Sensor/RConn1
  Voltage Sensor/LConn1 -- +/RConn1

== system inverter_switching_GridFollowing_StudentVersion/Subsystem2 ==
  Current Sensor : fl_lib/Electrical/Electrical Sensors/Current Sensor
  PS-Simulink Converter : nesl_utility/PS-Simulink Converter  PhysicalDomain=network_engine_domain  SubClassName=ps_output  LeftPortType=input  RightPortType=output  PseudoPeriodic=off  Frequencies=[]  VectorFormat=inherit  Unit=inherit  AffineConversion=off
  + : PMIOPort  Side=Left
  - : PMIOPort  Port=2  Side=Right
  i : Outport
  wires:
  PS-Simulink Converter/1 -> i/1
  connections:
  PS-Simulink Converter/LConn1 -- Current Sensor/RConn1
  Current Sensor/LConn1 -- +/RConn1
  Current Sensor/RConn2 -- -/RConn1

== system inverter_switching_GridFollowing_StudentVersion/Subsystem3 ==
  PS-Simulink Converter : nesl_utility/PS-Simulink Converter  PhysicalDomain=network_engine_domain  SubClassName=ps_output  LeftPortType=input  RightPortType=output  PseudoPeriodic=off  Frequencies=[]  VectorFormat=inherit  Unit=inherit  AffineConversion=off
  Voltage Sensor : fl_lib/Electrical/Electrical Sensors/Voltage Sensor
  + : PMIOPort  Side=Left
  - : PMIOPort  Port=2  Side=Right
  V : Outport
  wires:
  PS-Simulink Converter/1 -> V/1
  connections:
  Voltage Sensor/RConn2 -- -/RConn1
  PS-Simulink Converter/LConn1 -- Voltage Sensor/RConn1
  Voltage Sensor/LConn1 -- +/RConn1

== system inverter_switching_GridFollowing_StudentVersion/Subsystem4 ==
  PS-Simulink Converter : nesl_utility/PS-Simulink Converter  PhysicalDomain=network_engine_domain  SubClassName=ps_output  LeftPortType=input  RightPortType=output  PseudoPeriodic=off  Frequencies=[]  VectorFormat=inherit  Unit=inherit  AffineConversion=off
  Voltage Sensor : fl_lib/Electrical/Electrical Sensors/Voltage Sensor
  + : PMIOPort  Side=Left
  - : PMIOPort  Port=2  Side=Right
  V : Outport
  wires:
  PS-Simulink Converter/1 -> V/1
  connections:
  Voltage Sensor/LConn1 -- +/RConn1
  PS-Simulink Converter/LConn1 -- Voltage Sensor/RConn1
  Voltage Sensor/RConn2 -- -/RConn1

== system inverter_switching_GridFollowing_StudentVersion/Subsystem5 ==
  PS-Simulink Converter : nesl_utility/PS-Simulink Converter  PhysicalDomain=network_engine_domain  SubClassName=ps_output  LeftPortType=input  RightPortType=output  PseudoPeriodic=off  Frequencies=[]  VectorFormat=inherit  Unit=inherit  AffineConversion=off
  Voltage Sensor : fl_lib/Electrical/Electrical Sensors/Voltage Sensor
  + : PMIOPort  Side=Left
  - : PMIOPort  Port=2  Side=Right
  V : Outport
  wires:
  PS-Simulink Converter/1 -> V/1
  connections:
  Voltage Sensor/LConn1 -- +/RConn1
  PS-Simulink Converter/LConn1 -- Voltage Sensor/RConn1
  Voltage Sensor/RConn2 -- -/RConn1

== system inverter_switching_GridFollowing_StudentVersion/Subsystem6 ==
  PS-Simulink Converter : nesl_utility/PS-Simulink Converter  PhysicalDomain=network_engine_domain  SubClassName=ps_output  LeftPortType=input  RightPortType=output  PseudoPeriodic=off  Frequencies=[]  VectorFormat=inherit  Unit=inherit  AffineConversion=off
  Voltage Sensor : fl_lib/Electrical/Electrical Sensors/Voltage Sensor
  + : PMIOPort  Side=Left
  - : PMIOPort  Port=2  Side=Right
  V : Outport
  wires:
  PS-Simulink Converter/1 -> V/1
  connections:
  Voltage Sensor/RConn2 -- -/RConn1
  PS-Simulink Converter/LConn1 -- Voltage Sensor/RConn1
  Voltage Sensor/LConn1 -- +/RConn1

== system inverter_switching_GridFollowing_StudentVersion/Subsystem7 ==
  X_ac : Inport
  X_bc : Inport  Port=2
  Gain : Gain  Gain=T32*T32'  Multiplication=Matrix(K*u)
  Mux : Mux  Inputs=3
  X_abc : Outport
  wires:
  X_ac/1 -> Mux/1
  X_bc/1 -> Mux/2
  Mux/1 -> Gain/1
  Gain/1 -> X_abc/1

== system inverter_switching_GridFollowing_StudentVersion/Subsystem8 ==
  X_ac : Inport
  X_bc : Inport  Port=2
  Gain : Gain  Gain=T32*T32'  Multiplication=Matrix(K*u)
  Mux : Mux  Inputs=3
  X_abc : Outport
  wires:
  Gain/1 -> X_abc/1
  Mux/1 -> Gain/1
  X_bc/1 -> Mux/2
  X_ac/1 -> Mux/1

== system inverter_switching_GridFollowing_StudentVersion/Subsystem9 ==
  Current Sensor : fl_lib/Electrical/Electrical Sensors/Current Sensor
  PS-Simulink Converter : nesl_utility/PS-Simulink Converter  PhysicalDomain=network_engine_domain  SubClassName=ps_output  LeftPortType=input  RightPortType=output  PseudoPeriodic=off  Frequencies=[]  VectorFormat=inherit  Unit=inherit  AffineConversion=off
  + : PMIOPort  Side=Left
  - : PMIOPort  Port=2  Side=Right
  i : Outport
  wires:
  PS-Simulink Converter/1 -> i/1
  connections:
  Current Sensor/RConn2 -- -/RConn1
  Current Sensor/LConn1 -- +/RConn1
  PS-Simulink Converter/LConn1 -- Current Sensor/RConn1

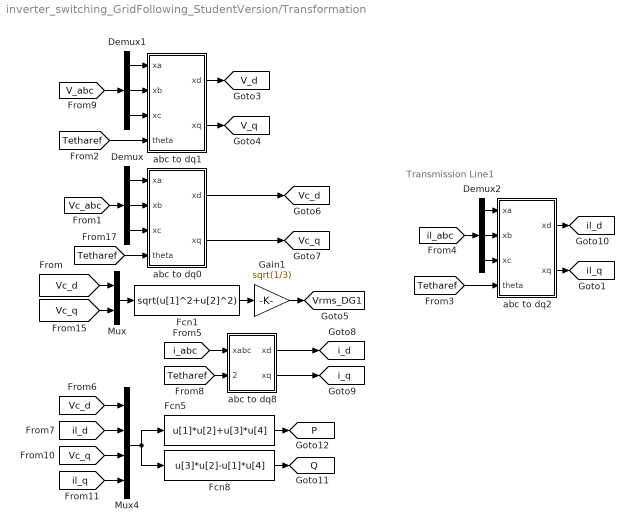
== system inverter_switching_GridFollowing_StudentVersion/Transformation ==
  note: Transmission Line1
  Demux : Demux  Outputs=3
  Demux1 : Demux  Outputs=3
  Demux2 : Demux  Outputs=3
  Fcn1 : Fcn  Expr=sqrt(u[1]^2+u[2]^2)
  Fcn5 : Fcn  Expr=u[1]*u[2]+u[3]*u[4]
  Fcn8 : Fcn  Expr=u[3]*u[2]-u[1]*u[4]
  Gain1 : Gain  Gain=sqrt(1/3)
  Mux : Mux  Inputs=2
  Mux4 : Mux
  abc to dq0 : Subsystem
  abc to dq1 : Subsystem
  abc to dq2 : Subsystem
  abc to dq8 : Subsystem
  tag scope: P=global, Q=global, V_d=global, V_q=global, Vc_d=global, Vc_q=global, Vrms_DG1=global, i_d=global, i_q=global, il_d=global, il_q=global
  wires:
  Mux4/1 -> Fcn8/1, Fcn5/1
  [Tetharef] -> abc to dq0/4(theta)
  Demux2/3 -> abc to dq2/3(xc)
  Demux2/2 -> abc to dq2/2(xb)
  Demux2/1 -> abc to dq2/1(xa)
  [il_abc] -> Demux2/1
  [Tetharef] -> abc to dq2/4(theta)
  [il_d] -> Mux4/2
  [il_q] -> Mux4/4
  [Vc_d] -> Mux4/1
  [Vc_q] -> Mux4/3
  Fcn5/1 -> [P]
  Fcn8/1 -> [Q]
  abc to dq2/1(xd) -> [il_d]
  abc to dq2/2(xq) -> [il_q]
  abc to dq0/1(xd) -> [Vc_d]
  abc to dq0/2(xq) -> [Vc_q]
  Gain1/1 -> [Vrms_DG1]
  Fcn1/1 -> Gain1/1
  Mux/1 -> Fcn1/1
  [Vc_d] -> Mux/1
  [Vc_q] -> Mux/2
  abc to dq8/2(xq) -> [i_q]
  abc to dq8/1(xd) -> [i_d]
  [Tetharef] -> abc to dq8/2(theta)
  [i_abc] -> abc to dq8/1(xabc)
  Demux/1 -> abc to dq0/1(xa)
  Demux/2 -> abc to dq0/2(xb)
  Demux/3 -> abc to dq0/3(xc)
  [Vc_abc] -> Demux/1
  Demux1/2 -> abc to dq1/2(xb)
  Demux1/3 -> abc to dq1/3(xc)
  Demux1/1 -> abc to dq1/1(xa)
  [V_abc] -> Demux1/1
  [Tetharef] -> abc to dq1/4(theta)
  abc to dq1/1(xd) -> [V_d]
  abc to dq1/2(xq) -> [V_q]

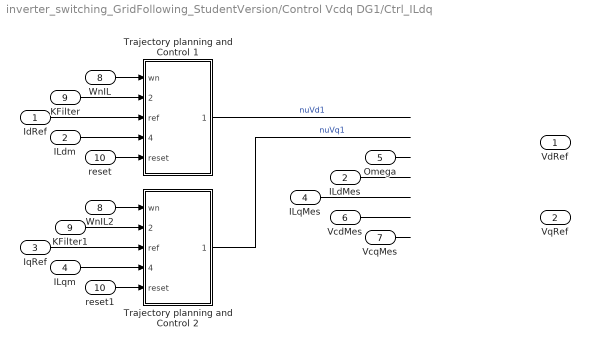
== system inverter_switching_GridFollowing_StudentVersion/Control Vcdq DG1/Ctrl_ILdq ==
  IdRef : Inport
  ILdm : Inport  Port=2
  IqRef : Inport  Port=3
  ILqm : Inport  Port=4
  Omega : Inport  Port=5
  VcdMes : Inport  Port=6
  VcqMes : Inport  Port=7
  WnIL : Inport  Port=8
  KFilter : Inport  Port=9
  reset : Inport  Port=10
  ILdMes : InportShadow  Port=2
  ILqMes : InportShadow  Port=4
  KFilter1 : InportShadow  Port=9
  Trajectory planning and Control 1 : Subsystem
  Trajectory planning and Control 2 : Subsystem
  WnIL2 : InportShadow  Port=8
  reset1 : InportShadow  Port=10
  VdRef : Outport
  VqRef : Outport  Port=2
  wires:
  Omega/1 -> ?
  ILdMes/1 -> ?
  ILqMes/1 -> ?
  VcqMes/1 -> ?
  VcdMes/1 -> ?
  ? -> VqRef/1
  ? -> VdRef/1
  Trajectory planning and Control 2/1(nuVd2) -> ?  "nuVq1"
  Trajectory planning and Control 1/1(nuVd2) -> ?  "nuVd1"
  KFilter1/1 -> Trajectory planning and Control 2/2(CoefFilter)
  WnIL2/1 -> Trajectory planning and Control 2/1(wn)
  KFilter/1 -> Trajectory planning and Control 1/2(CoefFilter)
  WnIL/1 -> Trajectory planning and Control 1/1(wn)
  reset/1 -> Trajectory planning and Control 1/5(reset)
  ILdm/1 -> Trajectory planning and Control 1/4(Measure)
  IdRef/1 -> Trajectory planning and Control 1/3(ref)
  IqRef/1 -> Trajectory planning and Control 2/3(ref)
  ILqm/1 -> Trajectory planning and Control 2/4(Measure)
  reset1/1 -> Trajectory planning and Control 2/5(reset)

== system inverter_switching_GridFollowing_StudentVersion/PLL/PLL ==
  vcq1 : Inport
  Vrms : Inport  Port=2
  Reset : Inport  Port=3
  Divide : Product  Inputs=*/
  Gain2 : Gain  Gain=sqrt(3)
  Gain3 : Gain  Gain=Kpll2
  Integrator : Integrator  ExternalReset=level  InitialCondition=wrated
  Integrator1 : Integrator  ExternalReset=level
  Reset1 : InportShadow  Port=3
  Transfer Fcn : TransferFcn  Numerator=[T1 1]  Denominator="[T2  1]"
  wpll : Outport
  theta_pll : Outport  Port=2
  wires:
  Divide/1 -> Gain3/1
  Transfer Fcn/1 -> Integrator/1
  Gain2/1 -> Divide/2
  Integrator/1 -> wpll/1, Integrator1/1
  Integrator1/1 -> theta_pll/1
  Gain3/1 -> Transfer Fcn/1
  Reset/1 -> Integrator/2
  Vrms/1 -> Gain2/1
  Reset1/1 -> Integrator1/2
  vcq1/1 -> Divide/1
